simulink model "CCCV"  (R2026a)
settings: Solver=VariableStepAuto  StopTime=15000  AbsTol=1e-3  EnableMultiTasking=on
libraries: fl_lib x8, nesl_utility x4, THERMALBattery_lib x1
settings Model: Creator=Soliana Hadera  LastModifiedBy=Soliana Hadera
settings SimscapeCC: SimscapeNominalValues="[{\"value\":\"1\",\"unit\":\"A\"},{\"value\":\"1\",\"unit\":\"bar\"},{\"value\":\"1\",\"unit\":\"cm^2\"},{\"value\":\"1\",\"unit\":\"cm^3/s\"},{\"value\":\"1\",\"unit\":\"kJ/kg\"},{\"value\":\"1\",\"unit\":\"kW\"},{\"value\":\"1\",\"unit\":\"l\"},{\"value\":\"1\",\"unit\":\"N\"},{\"value\":\"1\",\"unit\":\"N*m\"},{\"value\":\"1\",\"unit\":\"V\"}]"

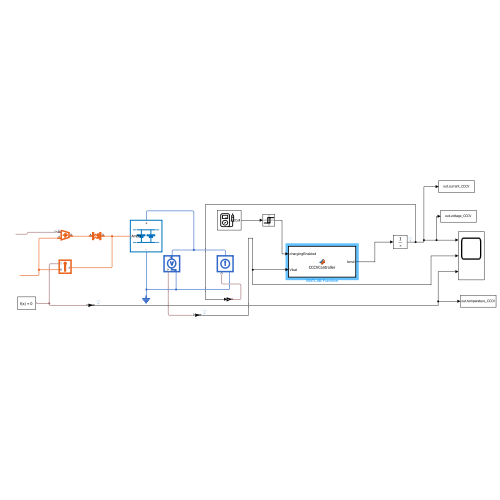
[thumbnail: Simulink's stored preview of the top-level diagram]
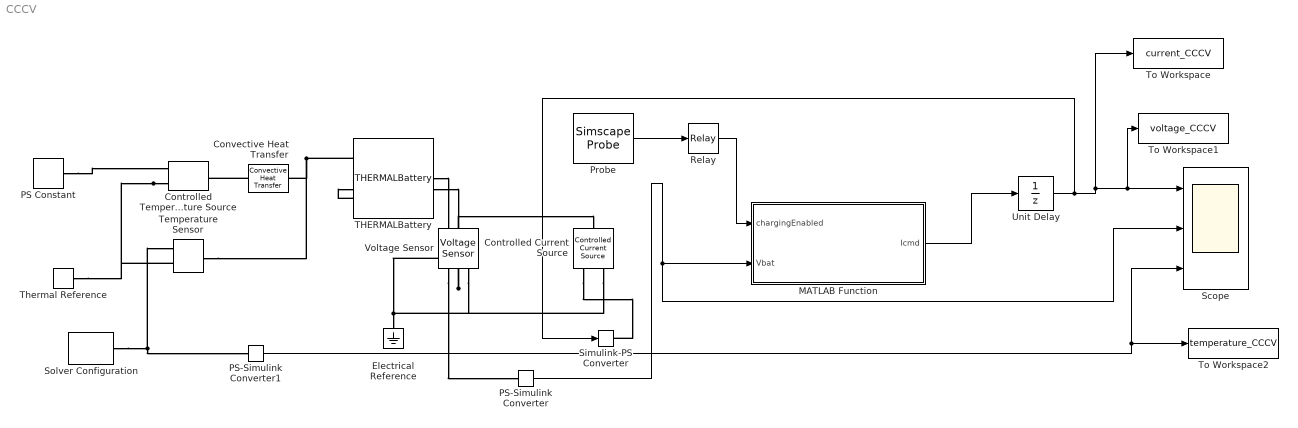
== system CCCV ==
  Controlled Temperature Source : fl_lib/Thermal/Thermal Sources/Controlled Temperature Source
  Controlled Current Source : fl_lib/Electrical/Electrical Sources/Controlled Current Source
  Convective Heat Transfer : fl_lib/Thermal/Thermal Elements/Convective Heat Transfer  thermal_type=foundation.enum.constant_variable.constant  area=0.0042 m^2  heat_tr_coeff=20 W/(K*m^2)  min_heat_tr_coeff=1e-3 W/(K*m^2)  T_specify=off  T_priority=None  T=0 K  T_nominal_specify=off  T_nominal_value=1  T_nominal_unit=K  Q_specify=off  Q_priority=None  Q=0 W  Q_nominal_specify=off  Q_nominal_value=1  Q_nominal_unit=W
  Electrical Reference : fl_lib/Electrical/Electrical Elements/Electrical Reference
  MATLAB Function : MATLAB Function  TreatAsAtomicUnit=on
  PS Constant : fl_lib/Physical Signals/Sources/PS Constant  constant=298.15
  PS-Simulink Converter : nesl_utility/PS-Simulink Converter  PhysicalDomain=network_engine_domain  SubClassName=ps_output  LeftPortType=input  RightPortType=output  PseudoPeriodic=off  Frequencies=[]  VectorFormat=inherit  Unit=inherit  AffineConversion=off
  PS-Simulink Converter1 : nesl_utility/PS-Simulink Converter  PhysicalDomain=network_engine_domain  SubClassName=ps_output  LeftPortType=input  RightPortType=output  PseudoPeriodic=off  Frequencies=[]  VectorFormat=inherit  Unit=inherit  AffineConversion=off
  Probe : SimscapeProbe  BoundBlock=46  Variables="{\"socCell\":{\"Probing\":\"ON\"}}"
  Relay : Relay  OnSwitchValue=.9  OffSwitchValue=0.2  OnOutputValue=0  OffOutputValue=1
  Scope : Scope  NumInputPorts=3
      settings: ActiveDisplayYMinimum=-1.8608777545548596  ActiveDisplayYMaximum=1.8328426436913323  YLabel=Current (A)
  Simulink-PS Converter : nesl_utility/Simulink-PS Converter  PhysicalDomain=network_engine_domain  SubClassName=ps_input  LeftPortType=input  RightPortType=output  PseudoPeriodic=off  Frequencies=[]  NoiseDistribution=none  NoiseParameters=[]  Unit=1  AffineConversion=off  FilteringAndDerivatives=provide  SimscapeFilterOrder=1  InputFilterTimeConstant=0.001  UdotUserProvided=0
  Solver Configuration : nesl_utility/Solver Configuration  PhysicalDomain=network_engine_domain  SubClassName=solver  LeftPortType=input  RightPortType=generic  Tones=[]  Harmonics=[]  SimulateNoise=off  Profile=off  UseLocalSampling=off  EnableSwitchedLinearOptims=on  FrequencyDomain=off  UseCCode=off  RelTol=0.001  AbsTol=0.001  MinStep=1e-09  ToWorkspace=off  RevertToSquareIcSolve=off  NumHomotopyIterations=100  PhasorMode=off  PhasorModeNumHarmonics=1  ConsistencySolver=NEWTON_XTOL_AFTER_FTOL  CanonicalOrdering=CANONICAL  OptimizeIntermediates=OPTIMIZED  IndexReductionMethod=DerivativeReplacement  DoDC=off  ResidualTolerance=1e-09  ConsistencyTolSource=GLOBAL  ConsistencyAbsTol=0.001  ConsistencyRelTol=0.001  ConsistencyTolFactor=0.001  UseLocalSolver=off  LocalSolverChoice=NE_BACKWARD_EULER_ADVANCER  ResolveIndetEquations=on  FunctionEvalNumThread=1  LocalSolverSampleTime=0.001  DoFixedCost=off  MaxNonlinIter=3  MaxModeIter=2  ComputeImpulses=off  ImpulseIterations=2  LinearAlgebra=auto  LinearAlgebraNumThread=0  EquationFormulation=NE_TIME_EF  DelaysMemoryBudget=1024  AutomaticFiltering=on  FilteringTimeConstant=0.001  PartitionStorageMethod=AS_NEEDED  PartitionMemoryBudget=1024  PartitionMethod=ROBUST  MultibodyUseLocalSolver=off  MultibodyLocalSolverChoice=ODE1  MultibodyLocalSolverSampleTime=0.001
  THERMALBattery : THERMALBattery_lib/THERMALBattery  BatteryCapacityCell=1.1 A*hr  ExtrapolationMethodCell=simscape.enum.extrapolation.nearest  SOCBreakpointsCell=[0, .1, .25, .5, .75, .9, 1]  TemperatureBreakpointsCell=[278, 293, 313] K  OpenCircuitVoltageThermalCell=|  VoltageRangeCell=[0, inf] V  ResistanceSOCBreakpointsCell=[0, .1, .25, .5, .75, .9, 1]  ResistanceTemperatureBreakpointsCell=[278, 293, 313] K  R0ThermalCell=[.0117, .0085, .009; .011, .0085, .009; .0114, .0087, .0092; .0107, .0082, .0088; .0107, .0083, .0091; .0113, .0085, .0089; .0116, .0085, .0089] Ohm  BatteryThermalMassCell=35 J/K  AmbientResistance=25 K/W  socCell_specify=on  socCell_priority=High  socCell=0.5  socCell_nominal_specify=off  socCell_nominal_value=1  socCell_nominal_unit=1  batteryVoltage_specify=off  batteryVoltage_priority=None  batteryVoltage=0 V  batteryVoltage_nominal_specify=off  batteryVoltage_nominal_value=1  batteryVoltage_nominal_unit=V  batteryCurrent_specify=off  batteryCurrent_priority=None  batteryCurrent=0 A  batteryCurrent_nominal_specify=off  batteryCurrent_nominal_value=1  batteryCurrent_nominal_unit=A  numCycles_specify=off  numCycles_priority=High  numCycles=0  numCycles_nominal_specify=off  numCycles_nominal_value=1  numCycles_nominal_unit=1  batteryTemperature_specify=off  batteryTemperature_priority=High  batteryTemperature=298.15 K  batteryTemperature_nominal_specify=off  batteryTemperature_nominal_value=1  batteryTemperature_nominal_unit=K  vParallelAssembly_specify=off  vParallelAssembly_priority=None  vParallelAssembly=0 V  vParallelAssembly_nominal_specify=off  vParallelAssembly_nominal_value=1  vParallelAssembly_nominal_unit=V  socParallelAssembly_specify=off  socParallelAssembly_priority=None  socParallelAssembly=1  socParallelAssembly_nominal_specify=off  socParallelAssembly_nominal_value=1  socParallelAssembly_nominal_unit=1
      | [ 2.50 2.50 2.50;
      | 3.05 3.05 3.05;
      | 3.22 3.22 3.22;
      | 3.29 3.29 3.29;
      | 3.32 3.32 3.32;
      | 3.36 3.36 3.36;
      | 3.40 3.40 3.40] V
  Temperature Sensor : fl_lib/Thermal/Thermal Sensors/Temperature Sensor  temperature_measure=foundation.enum.MeasurementReference.difference
  Thermal Reference : fl_lib/Thermal/Thermal Elements/Thermal Reference
  To Workspace : ToWorkspace  VariableName=current_CCCV  SaveFormat=Timeseries  SampleTime=-1
  To Workspace1 : ToWorkspace  VariableName=voltage_CCCV  SaveFormat=Timeseries  SampleTime=-1
  To Workspace2 : ToWorkspace  VariableName=temperature_CCCV  SaveFormat=Timeseries  SampleTime=-1
  Unit Delay : UnitDelay  SampleTime=-1
  Voltage Sensor : fl_lib/Electrical/Electrical Sensors/Voltage Sensor
  wires:
  PS-Simulink Converter1/1 -> To Workspace2/1, Scope/3
  Relay/1 -> MATLAB Function/1(chargingEnabled)
  Unit Delay/1 -> Simulink-PS Converter/1, To Workspace/1, To Workspace1/1, Scope/1
  PS-Simulink Converter/1 -> MATLAB Function/2(Vbat), Scope/2
  MATLAB Function/1(Icmd) -> Unit Delay/1
  Probe/1 -> Relay/1
  connections:
  Solver Configuration/RConn1 -- Temperature Sensor/RConn2 -- PS-Simulink Converter1/LConn1
  THERMALBattery/LConn1 -- Temperature Sensor/LConn1 -- Convective Heat Transfer/RConn1
  THERMALBattery/RConn1 -- Controlled Current Source/RConn2 -- Voltage Sensor/RConn2 -- Electrical Reference/LConn1
  THERMALBattery/LConn2 -- Controlled Current Source/LConn1 -- Voltage Sensor/LConn1
  Controlled Temperature Source/RConn2 -- Thermal Reference/LConn1 -- Temperature Sensor/RConn1
  Convective Heat Transfer/LConn1 -- Controlled Temperature Source/LConn1
  Controlled Current Source/RConn1 -- Simulink-PS Converter/RConn1
  PS Constant/RConn1 -- Controlled Temperature Source/RConn1
  Voltage Sensor/RConn1 -- PS-Simulink Converter/LConn1

== matlab function CCCV/MATLAB Function ==
  data: chargingEnabled input; Icmd output; Vbat input
function Icmd = CCCVController(chargingEnabled, Vbat)

Icharge = 1.5;      % A
Idischarge = 1.1;   % A
Vtarget = 3.60;     % V
Kp = 10;

if chargingEnabled

    % Constant-current charging
    if Vbat < 3.50
        Icmd = Icharge;

        % Constant-voltage charging
    else
        Icmd = Kp*(Vtarget - Vbat);

        % Limit charging current
        Icmd = min(max(Icmd,0),Icharge);
    end

else

    % Constant-current discharge
    Icmd = -Idischarge;

end
